simulink model "testrig_half_car_spla_s2laf_au"  (R2023a)
settings: Solver=ode23t  StartTime=0.0  StopTime=192  MaxStep=0.05  RelTol=1e-3  AbsTol=1e-3  EnableMultiTasking=on
PostLoadFcn:
  | sm_car_load_vehicle_data(bdroot,'220');
  | 
  | Vehicle.Chassis.SuspA1.Linkage.Upper_Arm_to_Subframe.class.Value  = 'Rigid_1Rev';
  | Vehicle.Chassis.SuspA1.Linkage.LowerArmF_to_Subframe.class.Value  = 'Rigid_UJ';
  | Vehicle.Chassis.SuspA1.Linkage.LowerArmR_to_Subframe.class.Value  = 'Rigid_UJ';
  | Vehicle.Chassis.SuspA1.AntiRollBar.SubframeConnection.class.Value = 'Rigid_1Rev';
  | 
  | Maneuver = sm_car_maneuverdata_knc(0.22,-0.15,0.01,1.0,0.10,500,1200,1200);
  | Vehicle = sm_car_vehcfg_checkConfig(Vehicle);
  | Visual = sm_car_param_visual('default');
undefined symbols (not defined in the file or in its folder): X, Y, Z
libraries: sm_lib x14, sm_car_testrig_utilities_lib x4, nesl_utility x4, fl_lib x4, Damper_Element x2, Linkage_SpLA_S2LAF_AU x2, Spring_Element x2, Suspension_Utilities x2, AntiRollBar_Droplink_Rod x1
CloseFcn:
  | clear simlog_sm_car_testrig_quarter_car
  | clear logsout_sm_car_testrig_quarter_car
Description:
  | Half Car Testrig, Pullrod
  | 
  | Copyright 2021-2024 The MathWorks, Inc.
settings Model: Creator=smiller  LastModifiedBy=smiller
settings SolverCC: AutoScaleAbsTol=off  AlgebraicLoopSolver=TrustRegion
settings DataIOCC: LimitDataPoints=on  MaxDataPoints=10000  ReturnWorkspaceOutputs=off  SignalLoggingName=logsout_sm_car_testrig_quarter_car
settings OptimizationCC: LifeSpan=inf
settings DebuggingCC: UnconnectedInputMsg=warning  UnconnectedOutputMsg=warning  UnconnectedLineMsg=warning  AllowSymbolicDim=off  SFUnexpectedBacktrackingDiag=warning  SFNoUnconditionalDefaultTransitionDiag=warning  SFExecutionAtInitializationDiag=none  ArithmeticOperatorsInVariantConditions=warning
settings ModelReferenceCC: EnableRefExpFcnMdlSchedulingChecks=on
settings SFSimCC: SimUseLocalCustomCode=off  CustomCodeUndefinedFunction=UseInterfaceOnly
settings RTWCC: RTWUseLocalCustomCode=off
settings CodeAppCC: StateflowObjectComments=on
settings GRTTargetCC: TargetLangStandard=C89/C90 (ANSI)
settings ConfigComp: CovMetricSettings=dw  CovSaveCumulativeToWorkspaceVar=on  CovSaveSingleToWorkspaceVar=on  CovExternalEMLEnable=off  CovSFcnEnable=off
settings SimscapeCC: SimscapeLogType=all  SimscapeLogSimulationStatistics=on  SimscapeLogName=simlog_sm_car_testrig_quarter_car  SimscapeLogLimitData=off  SimscapeLogDataHistory=10000  SimscapeOperatingPoint=op
settings DiagnosticsConfigSet: SimMechanicsUnconnectedFramePorts=none
settings ExplorerConfigSet: InternalSimMechanicsExplorerSettings="<ExplorerConfiguration><canonicalview>default</canonicalview><AnimationSetting><BasePlaybackSpeed>1.0</BasePlaybackSpeed><PlaybackSpeedFactor>16.0</PlaybackSpeedFactor></AnimationSetting><TilePanel><TileInfo><Tiles Columns=\"1\" Count=\"1\" Rows=\"1\"><Column Weight=\"1\"/><Row Weight=\"1\"/><Tile Height=\"1\" Width=\"1\" X=\"0\" Y=\"0\"/></Tiles></TileInfo><SceneInfo><SceneViewer><BGColor><R>1</R><G>1</G><B>1</B></BGColor><Camera><DoPerspective>off</DoPerspective><Position><X>0.571928528858414942</X><Y>-0.579111562749420217</Y><Z>0.83606068842340453</Z></Position><Center><X>-0.00542174033121090027</X><Y>-0.00176129355979437463</Y><Z>0.258710419233778688</Z></Center><Up><X>-0.408248290463863073</X><Y>0.408248290463863073</Y><Z>0.816496580927726145</Z></Up><ViewLimDist>1</ViewLimDist><YLim>0.718679582981457732</YLim><XLim>0.891323281686500546</XLim></Camera></SceneViewer></SceneInfo></TilePanel><MechEditorPanel><Cameras/><GfxPanelCameraMap/><VideoCreator><PlaybackSpeedRatio>1.0</PlaybackSpeedRatio><FrameRate>30</FrameRate><VideoFormat>Motion JPEG AVI</VideoFormat><FrameSize>auto</FrameSize></VideoCreator></MechEditorPanel></ExplorerConfiguration>"

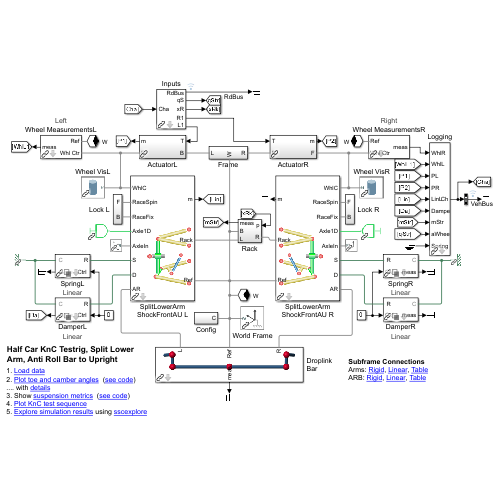
[thumbnail: Simulink's stored preview of the top-level diagram]
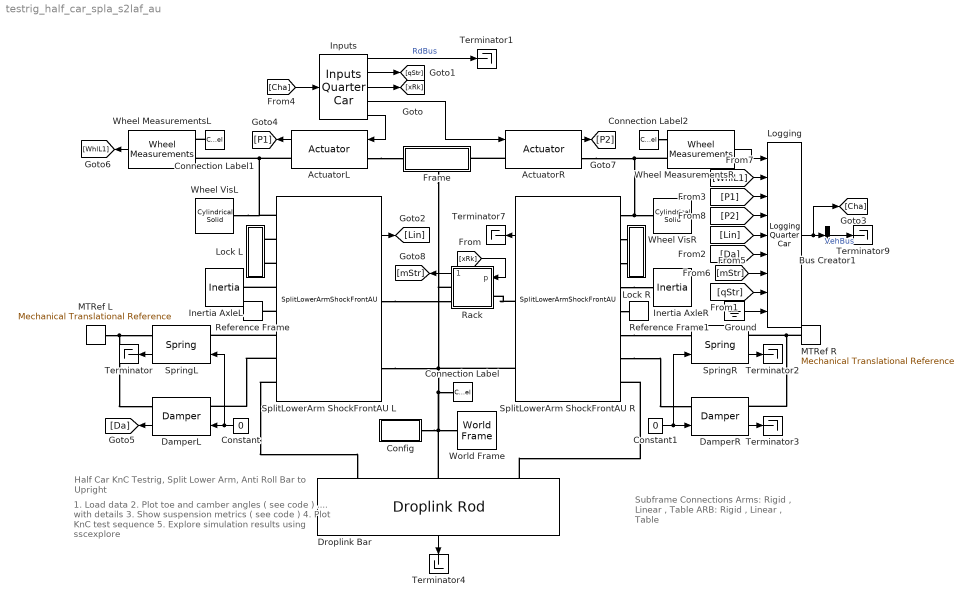
== system testrig_half_car_spla_s2laf_au ==
  note: Subframe Connections
      | Arms: Rigid , Linear , Table
      | ARB: Rigid , Linear , Table
  note: Half Car KnC Testrig, Split Lower
      | Arm, Anti Roll Bar to Upright
  note: 1. Load data
      | 2. Plot toe and camber angles ( see code )
      | .... with details
      | 3. Show suspension metrics ( see code )
      | 4. Plot KnC test sequence
      | 5. Explore simulation results using sscexplore
  ActuatorL : sm_car_testrig_utilities_lib/Actuator  SystemSampleTime=-1  VariantActivationTime=update diagram  Latency=0  AutoFrameSizeCalculation=off
  ActuatorR : sm_car_testrig_utilities_lib/Actuator  SystemSampleTime=-1  VariantActivationTime=update diagram  Latency=0  AutoFrameSizeCalculation=off
  Bus Creator1 : BusCreator  Inputs=1
  Config : Subsystem
  Connection Label : ConnectionLabel  Label=W
  Connection Label1 : ConnectionLabel  Label=W
  Connection Label2 : ConnectionLabel  Label=W
  Constant : Constant  Value=0
  Constant1 : Constant  Value=0
  DamperL : Damper_Element/Damper  VariantControl=Variant1  LabelModeActiveChoice=Linear  Damper=Vehicle.Chassis.Damper.Axle1  VariantLabel=Vehicle.Chassis.Damper.Axle1.class.Value
      settings: AttributesFormatString=%<ActiveVariant>
  DamperR : Damper_Element/Damper  VariantControl=Variant1  LabelModeActiveChoice=Linear  Damper=Vehicle.Chassis.Damper.Axle1  VariantLabel=Vehicle.Chassis.Damper.Axle1.class.Value
      settings: AttributesFormatString=%<ActiveVariant>
  Droplink Bar : AntiRollBar_Droplink_Rod/Droplink Rod  VariantControl=Variant1  hp_rod=Vehicle.Chassis.SuspA1.AntiRollBar.sSuspension.Value  hp_out=Vehicle.Chassis.SuspA1.AntiRollBar.sOutboard.Value  hp_in=Vehicle.Chassis.SuspA1.AntiRollBar.sInboard.Value  hp_mount_subframe=Vehicle.Chassis.SuspA1.AntiRollBar.sMount.Value  rotYAxis=Vehicle.Chassis.SuspA1.AntiRollBar.qUniversal.Value  SubframeConnection=Vehicle.Chassis.SuspA1.AntiRollBar.SubframeConnection  k=Vehicle.Chassis.SuspA1.AntiRollBar.k.Value  d=Vehicle.Chassis.SuspA1.AntiRollBar.d.Value  m=Vehicle.Chassis.SuspA1.AntiRollBar.m.Value  clr_solid=Visual.AntiRollBar.clr  opc_solid=Visual.part.opc  rad_solid=Visual.AntiRollBar.rad  clr_hp=Visual.hp.clr  opc_hp=Visual.hp.opc  rad_hp=Visual.hp.rad
  Frame : Subsystem
      settings: PortSchema="{\"entries\":[{\"content\":{\"sides\":[{\"content\":{\"connectorIds\":[\"LConn1\"]},\"type\":\"ConnectorPlacement.EquallySpacedRectSide\",\"uuid\":\"4d1860d1-8382-4b55-85c2-09349d56bb16\"},{\"content\":{\"connectorIds\":[\"RConn1\"],\"side\":\"RIGHT\"},\"type\":\"ConnectorPlacement.EquallySpacedRectSide\",\"uuid\":\"4e90683f-4b1a-48f4-aa4c-ab416257a32f\"},{\"content\":{\"connectorIds\":[],\"side\":\"TOP\"},\"type\":\"ConnectorPlacement.EquallySpacedRectSide\",\"uuid\":\"73ac831e-e43d-4cda-a295-19295eab84b4\"},{\"content\":{\"connectorIds\":[\"RConn2\"],\"side\":\"BOTTOM\"},\"type\":\"ConnectorPlacement.EquallySpacedRectSide\",\"uuid\":\"24788d71-0cf9-496d-9e47-2bd8b288be51\"}]},\"type\":\"ConnectorPlacement.EquallySpacedConnector\",\"uuid\":\"859ec081-8f6e-43e9-9a98-d438cbc0fcb8\"}],\"packageUris\":[\"http://schema.mathworks.com/mf0/Connector/R2020b\"],\"version\":\"1.0\"}"
  Ground : Ground
  Inertia AxleL : fl_lib/Mechanical/Rotational Elements/Inertia  inertia=0.01 kg*m^2  num_ports=foundation.enum.numPorts2.one  w_specify=on  w_priority=None  w=0 rad/s  w_nominal_specify=off  w_nominal_unit=rad/s  w_nominal_value=1  t_specify=off  t_priority=None  t=0 N*m  t_nominal_specify=off  t_nominal_unit=N*m  t_nominal_value=1
  Inertia AxleR : fl_lib/Mechanical/Rotational Elements/Inertia  inertia=0.01 kg*m^2  num_ports=foundation.enum.numPorts2.one  w_specify=on  w_priority=None  w=0 rad/s  w_nominal_specify=off  w_nominal_unit=rad/s  w_nominal_value=1  t_specify=off  t_priority=None  t=0 N*m  t_nominal_specify=off  t_nominal_unit=N*m  t_nominal_value=1
  Inputs : sm_car_testrig_utilities_lib/Inputs Quarter Car  popup_steering_input=On
  Lock L : Subsystem
  Lock R : Subsystem
  Logging : sm_car_testrig_utilities_lib/Logging Quarter Car
  MTRef L : fl_lib/Mechanical/Translational Elements/Mechanical Translational Reference
  MTRef R : fl_lib/Mechanical/Translational Elements/Mechanical Translational Reference
  Rack : Subsystem
  Reference Frame : sm_lib/Frames and Transforms/Reference Frame
  Reference Frame1 : sm_lib/Frames and Transforms/Reference Frame
  SplitLowerArm ShockFrontAU L : Linkage_SpLA_S2LAF_AU/SplitLowerArmShockFrontAU  VariantControl=SplitLowerArmShockFront  popup_leftRight=Left  hp_in_f_ua=Vehicle.Chassis.SuspA1.Linkage.UpperWishbone.sInboardF.Value  hp_in_r_ua=Vehicle.Chassis.SuspA1.Linkage.UpperWishbone.sInboardR.Value  hp_out_ua=Vehicle.Chassis.SuspA1.Linkage.UpperWishbone.sOutboard.Value  hp_in_f_la=Vehicle.Chassis.SuspA1.Linkage.LowerArmF.sInboard.Value  hp_in_r_la=Vehicle.Chassis.SuspA1.Linkage.LowerArmR.sInboard.Value  hp_out_f_la=Vehicle.Chassis.SuspA1.Linkage.LowerArmF.sOutboard.Value  hp_out_r_la=Vehicle.Chassis.SuspA1.Linkage.LowerArmR.sOutboard.Value  hp_upr_cg=Vehicle.Chassis.SuspA1.Linkage.Upright.sCG.Value  hp_upr_wc=Vehicle.Chassis.SuspA1.Linkage.Upright.sWheelCentre.Value  hp_upr_arb=Vehicle.Chassis.SuspA1.Linkage.Upright.sARB.Value  hp_in_rod=Vehicle.Chassis.SuspA1.Linkage.TrackRod.sInboard.Value  hp_upr_rod=Vehicle.Chassis.SuspA1.Linkage.TrackRod.sOutboard.Value  hp_spr_top=Vehicle.Chassis.SuspA1.Linkage.Shock.sTop.Value  hp_spr_bot=Vehicle.Chassis.SuspA1.Linkage.Shock.sBottom.Value  clr_hp=Visual.hp.clr  opc_hp=Visual.hp.opc  size_hp=Visual.hp.rad  Upper_Arm_to_Subframe=Vehicle.Chassis.SuspA1.Linkage.Upper_Arm_to_Subframe  ua_mass=Vehicle.Chassis.SuspA1.Linkage.UpperWishbone.m.Value  clr_ua=Visual.UpperArm.clr  opc_ua=Visual.part.opc  radius_ua=Visual.UpperArm.rad  LowerArmF_to_Subframe=Vehicle.Chassis.SuspA1.Linkage.LowerArmF_to_Subframe  LowerArmR_to_Subframe=Vehicle.Chassis.SuspA1.Linkage.LowerArmR_to_Subframe  laf_mass=Vehicle.Chassis.SuspA1.Linkage.LowerArmF.m.Value  lar_mass=Vehicle.Chassis.SuspA1.Linkage.LowerArmR.m.Value  clr_conn_la=Visual.hp.clr  opc_conn_la=Visual.hp.opc  size_conn_la=Visual.hp.rad  clr_laf=Visual.LowerArm.clr  opc_laf=Visual.part.opc  radius_laf=Visual.LowerArm.rad  clr_lar=Visual.LowerArm.clr  opc_lar=Visual.part.opc  radius_lar=Visual.LowerArm.rad  shock_pist_mass=Vehicle.Chassis.SuspA1.Linkage.Shock.mPiston.Value  shock_cyl_mass=Vehicle.Chassis.SuspA1.Linkage.Shock.mCylinder.Value  up_lim_bumpstop=Vehicle.Chassis.SuspA1.Linkage.Endstop.xMax.Value  low_lim_bumpstop=Vehicle.Chassis.SuspA1.Linkage.Endstop.xMin.Value  clr_conn_shock=Visual.hp.clr  opc_conn_shock=Visual.hp.opc  size_conn_shock=Visual.hp.rad  clr_shock_cyl=Visual.Shock.cyl.clr  opc_shock_cyl=Visual.part.opc  radius_shock_cyl=Visual.Shock.cyl.rad  clr_shock_piston=Visual.Shock.piston.clr  opc_shock_piston=Visual.part.opc  clr_shock_bumpstop=Visual.Shock.bumpstop.clr  opc_shock_bumpstop=Visual.part.opc  deadvol_len_shock_cyl=Visual.Shock.dead_length  piston_len_shock=Visual.Shock.piston.len  cyl_cap_len_shock=Visual.Shock.cap.len  bumpstop_len_shock=Visual.Shock.bumpstop.len  atoe=Vehicle.Chassis.SuspA1.Linkage.Upright.aToe.Value  acamber=Vehicle.Chassis.SuspA1.Linkage.Upright.aCamber.Value  upr_mass=Vehicle.Chassis.SuspA1.Linkage.Upright.m.Value  axle_len=Vehicle.Chassis.SuspA1.Linkage.Upright.xAxle.Value  axle_whlc_to_bearing=Vehicle.Chassis.SuspA1.Linkage.Upright.xWCtoBearing.Value  axle_mass=Vehicle.Chassis.SuspA1.Linkage.Upright.mAxle.Value  clr_conn_upr=Visual.hp.clr  opc_conn_upr=Visual.hp.opc  size_conn_upr=Visual.hp.rad  clr_upr=Visual.Upright.clr  opc_upr=Visual.part.opc  radius_upr=Visual.Upright.rad  clr_axle=Visual.Axle.clr  opc_axle=Visual.part.opc  radius_axle=Visual.Axle.rad  rod_mass=Vehicle.Chassis.SuspA1.Linkage.TrackRod.m.Value  clr_conn_rod=Visual.hp.clr  opc_conn_rod=Visual.hp.opc  size_conn_rod=Visual.hp.rad  clr_rod=Visual.TrackRod.clr  opc_rod=Visual.part.opc  radius_rod=Visual.TrackRod.rad  whl_init_spd_lr=Init.Axle1.nWheel.Value
  SplitLowerArm ShockFrontAU R : Linkage_SpLA_S2LAF_AU/SplitLowerArmShockFrontAU  VariantControl=SplitLowerArmShockFront  popup_leftRight=Right  hp_in_f_ua=Vehicle.Chassis.SuspA1.Linkage.UpperWishbone.sInboardF.Value  hp_in_r_ua=Vehicle.Chassis.SuspA1.Linkage.UpperWishbone.sInboardR.Value  hp_out_ua=Vehicle.Chassis.SuspA1.Linkage.UpperWishbone.sOutboard.Value  hp_in_f_la=Vehicle.Chassis.SuspA1.Linkage.LowerArmF.sInboard.Value  hp_in_r_la=Vehicle.Chassis.SuspA1.Linkage.LowerArmR.sInboard.Value  hp_out_f_la=Vehicle.Chassis.SuspA1.Linkage.LowerArmF.sOutboard.Value  hp_out_r_la=Vehicle.Chassis.SuspA1.Linkage.LowerArmR.sOutboard.Value  hp_upr_cg=Vehicle.Chassis.SuspA1.Linkage.Upright.sCG.Value  hp_upr_wc=Vehicle.Chassis.SuspA1.Linkage.Upright.sWheelCentre.Value  hp_upr_arb=Vehicle.Chassis.SuspA1.Linkage.Upright.sARB.Value  hp_in_rod=Vehicle.Chassis.SuspA1.Linkage.TrackRod.sInboard.Value  hp_upr_rod=Vehicle.Chassis.SuspA1.Linkage.TrackRod.sOutboard.Value  hp_spr_top=Vehicle.Chassis.SuspA1.Linkage.Shock.sTop.Value  hp_spr_bot=Vehicle.Chassis.SuspA1.Linkage.Shock.sBottom.Value  clr_hp=Visual.hp.clr  opc_hp=Visual.hp.opc  size_hp=Visual.hp.rad  Upper_Arm_to_Subframe=Vehicle.Chassis.SuspA1.Linkage.Upper_Arm_to_Subframe  ua_mass=Vehicle.Chassis.SuspA1.Linkage.UpperWishbone.m.Value  clr_ua=Visual.UpperArm.clr  opc_ua=Visual.part.opc  radius_ua=Visual.UpperArm.rad  LowerArmF_to_Subframe=Vehicle.Chassis.SuspA1.Linkage.LowerArmF_to_Subframe  LowerArmR_to_Subframe=Vehicle.Chassis.SuspA1.Linkage.LowerArmR_to_Subframe  laf_mass=Vehicle.Chassis.SuspA1.Linkage.LowerArmF.m.Value  lar_mass=Vehicle.Chassis.SuspA1.Linkage.LowerArmR.m.Value  clr_conn_la=Visual.hp.clr  opc_conn_la=Visual.hp.opc  size_conn_la=Visual.hp.rad  clr_laf=Visual.LowerArm.clr  opc_laf=Visual.part.opc  radius_laf=Visual.LowerArm.rad  clr_lar=Visual.LowerArm.clr  opc_lar=Visual.part.opc  radius_lar=Visual.LowerArm.rad  shock_pist_mass=Vehicle.Chassis.SuspA1.Linkage.Shock.mPiston.Value  shock_cyl_mass=Vehicle.Chassis.SuspA1.Linkage.Shock.mCylinder.Value  up_lim_bumpstop=Vehicle.Chassis.SuspA1.Linkage.Endstop.xMax.Value  low_lim_bumpstop=Vehicle.Chassis.SuspA1.Linkage.Endstop.xMin.Value  clr_conn_shock=Visual.hp.clr  opc_conn_shock=Visual.hp.opc  size_conn_shock=Visual.hp.rad  clr_shock_cyl=Visual.Shock.cyl.clr  opc_shock_cyl=Visual.part.opc  radius_shock_cyl=Visual.Shock.cyl.rad  clr_shock_piston=Visual.Shock.piston.clr  opc_shock_piston=Visual.part.opc  clr_shock_bumpstop=Visual.Shock.bumpstop.clr  opc_shock_bumpstop=Visual.part.opc  deadvol_len_shock_cyl=Visual.Shock.dead_length  piston_len_shock=Visual.Shock.piston.len  cyl_cap_len_shock=Visual.Shock.cap.len  bumpstop_len_shock=Visual.Shock.bumpstop.len  atoe=Vehicle.Chassis.SuspA1.Linkage.Upright.aToe.Value  acamber=Vehicle.Chassis.SuspA1.Linkage.Upright.aCamber.Value  upr_mass=Vehicle.Chassis.SuspA1.Linkage.Upright.m.Value  axle_len=Vehicle.Chassis.SuspA1.Linkage.Upright.xAxle.Value  axle_whlc_to_bearing=Vehicle.Chassis.SuspA1.Linkage.Upright.xWCtoBearing.Value  axle_mass=Vehicle.Chassis.SuspA1.Linkage.Upright.mAxle.Value  clr_conn_upr=Visual.hp.clr  opc_conn_upr=Visual.hp.opc  size_conn_upr=Visual.hp.rad  clr_upr=Visual.Upright.clr  opc_upr=Visual.part.opc  radius_upr=Visual.Upright.rad  clr_axle=Visual.Axle.clr  opc_axle=Visual.part.opc  radius_axle=Visual.Axle.rad  rod_mass=Vehicle.Chassis.SuspA1.Linkage.TrackRod.m.Value  clr_conn_rod=Visual.hp.clr  opc_conn_rod=Visual.hp.opc  size_conn_rod=Visual.hp.rad  clr_rod=Visual.TrackRod.clr  opc_rod=Visual.part.opc  radius_rod=Visual.TrackRod.rad  whl_init_spd_lr=Init.Axle1.nWheel.Value
  SpringL : Spring_Element/Spring  VariantControl=Variant1  LabelModeActiveChoice=Linear  Spring=Vehicle.Chassis.Spring.Axle1  VariantLabel=Vehicle.Chassis.Spring.Axle1.class.Value
      settings: AttributesFormatString=%<ActiveVariant>
  SpringR : Spring_Element/Spring  VariantControl=Variant1  LabelModeActiveChoice=Linear  Spring=Vehicle.Chassis.Spring.Axle1  VariantLabel=Vehicle.Chassis.Spring.Axle1.class.Value
      settings: AttributesFormatString=%<ActiveVariant>
  Terminator{,1..4,7,9} (7 alike) : Terminator
  Wheel MeasurementsL : Suspension_Utilities/Wheel Measurements  popup_leftRight=Left
      settings: AttributesFormatString=%<popup_leftRight>
  Wheel MeasurementsR : Suspension_Utilities/Wheel Measurements  popup_leftRight=Right
      settings: AttributesFormatString=%<popup_leftRight>
  Wheel VisL : sm_lib/Body Elements/Cylindrical Solid  GraphicAmbientColor=[0.15 0.15 0.15 1.0]  BasedOnType=Mass  CenterOfMass=[0 0 0]  CenterOfMassUnits=m  GraphicDiffuseColor=[0.5 0.5 0.5]  CylinderLength=Vehicle.Chassis.TireA1.tire_radius.Value*0.6  CylinderLengthUnits=m  CylinderRadius=Vehicle.Chassis.TireA1.tire_radius.Value  CylinderRadiusUnits=m  Density=1000  DensityUnits=kg/m^3  DoExposeReferenceFrame=on  GraphicEmissiveColor=[0.0 0.0 0.0 1.0]  ExportEntireGeometry=off  SerializedFrames=<Frames/>  MarkerShape=Sphere  MarkerSize=10  GraphicType=FromGeometry  InertiaType=CalculateFromGeometry  Mass=Vehicle.Chassis.TireA1.Mass.Value  MassUnits=kg  MomentsOfInertia=[1 1 1]  MomentsOfInertiaUnits=kg*m^2  GraphicOpacity=0.3  ProductsOfInertia=[0 0 0]  ProductsOfInertiaUnits=kg*m^2  GraphicShininess=75  GraphicSpecularColor=[0.5 0.5 0.5 1.0]  GraphicVisPropType=SimpleVisualProperties
  Wheel VisR : sm_lib/Body Elements/Cylindrical Solid  GraphicAmbientColor=[0.15 0.15 0.15 1.0]  BasedOnType=Mass  CenterOfMass=[0 0 0]  CenterOfMassUnits=m  GraphicDiffuseColor=[0.5 0.5 0.5]  CylinderLength=Vehicle.Chassis.TireA1.tire_radius.Value*0.6  CylinderLengthUnits=m  CylinderRadius=Vehicle.Chassis.TireA1.tire_radius.Value  CylinderRadiusUnits=m  Density=1000  DensityUnits=kg/m^3  DoExposeReferenceFrame=on  GraphicEmissiveColor=[0.0 0.0 0.0 1.0]  ExportEntireGeometry=off  SerializedFrames=<Frames/>  MarkerShape=Sphere  MarkerSize=10  GraphicType=FromGeometry  InertiaType=CalculateFromGeometry  Mass=Vehicle.Chassis.TireA1.Mass.Value  MassUnits=kg  MomentsOfInertia=[1 1 1]  MomentsOfInertiaUnits=kg*m^2  GraphicOpacity=0.3  ProductsOfInertia=[0 0 0]  ProductsOfInertiaUnits=kg*m^2  GraphicShininess=75  GraphicSpecularColor=[0.5 0.5 0.5 1.0]  GraphicVisPropType=SimpleVisualProperties
  World Frame : sm_lib/Frames and Transforms/World Frame
  wires:
  DamperL/1 -> [Da]
  Constant/1 -> SpringL/1, DamperL/1
  SpringL/1 -> Terminator/1
  [xRk] -> Rack/1(p)
  SpringR/1 -> Terminator2/1
  Constant1/1 -> SpringR/1, DamperR/1
  DamperR/1 -> Terminator3/1
  Droplink Bar/1 -> Terminator4/1
  ActuatorR/1 -> [P2]
  SplitLowerArm ShockFrontAU L/1 -> [Lin]
  SplitLowerArm ShockFrontAU R/1 -> Terminator7/1
  Wheel MeasurementsL/1 -> [WhlL1]
  [P1] -> Logging/3
  [Lin] -> Logging/5
  [WhlL1] -> Logging/2
  Bus Creator1/1 -> Terminator9/1  "VehBus"
  ActuatorL/1 -> [P1]
  [Cha] -> Inputs/1
  Inputs/5 -> ActuatorL/1
  Inputs/4 -> ActuatorR/1
  Inputs/2 -> [qStr]
  Inputs/3 -> [xRk]
  Inputs/1 -> Terminator1/1  "RdBus"
  Wheel MeasurementsR/1 -> Logging/1
  Logging/1 -> [Cha], Bus Creator1/1
  [Da] -> Logging/6
  [mStr] -> Logging/7
  [qStr] -> Logging/8
  Ground/1 -> Logging/9
  [P2] -> Logging/4
  Rack/1(meas) -> [mStr]
  connections:
  Wheel VisL/RConn1 -- SplitLowerArm ShockFrontAU L/LConn1 -- ActuatorL/RConn1 -- Wheel MeasurementsL/LConn2
  MTRef L/LConn1 -- SpringL/RConn1 -- DamperL/RConn1
  Config/RConn1 -- Droplink Bar/LConn2 -- World Frame/RConn1 -- Frame/RConn2 -- Rack/RConn1 -- SplitLowerArm ShockFrontAU R/RConn2 -- SplitLowerArm ShockFrontAU L/RConn2 -- Connection Label/LConn1
  SplitLowerArm ShockFrontAU L/LConn6 -- SpringL/LConn1
  SplitLowerArm ShockFrontAU L/LConn4 -- Inertia AxleL/LConn1
  SplitLowerArm ShockFrontAU L/LConn5 -- Reference Frame/RConn1
  SplitLowerArm ShockFrontAU L/LConn7 -- DamperL/LConn1
  SplitLowerArm ShockFrontAU L/RConn1 -- Rack/RConn2
  ActuatorR/RConn1 -- SplitLowerArm ShockFrontAU R/LConn1 -- Wheel VisR/RConn1 -- Wheel MeasurementsR/LConn2
  MTRef R/LConn1 -- DamperR/RConn1 -- SpringR/RConn1
  SplitLowerArm ShockFrontAU R/LConn4 -- Inertia AxleR/LConn1
  SplitLowerArm ShockFrontAU R/LConn6 -- SpringR/LConn1
  SplitLowerArm ShockFrontAU R/LConn5 -- Reference Frame1/RConn1
  SplitLowerArm ShockFrontAU R/LConn7 -- DamperR/LConn1
  SplitLowerArm ShockFrontAU L/LConn8 -- Droplink Bar/LConn1
  SplitLowerArm ShockFrontAU R/RConn1 -- Rack/LConn1
  SplitLowerArm ShockFrontAU R/LConn2 -- Lock R/LConn1
  SplitLowerArm ShockFrontAU R/LConn3 -- Lock R/LConn2
  SplitLowerArm ShockFrontAU L/LConn2 -- Lock L/LConn1
  SplitLowerArm ShockFrontAU L/LConn3 -- Lock L/LConn2
  ActuatorL/LConn1 -- Frame/LConn1
  ActuatorR/LConn1 -- Frame/RConn1
  Connection Label1/LConn1 -- Wheel MeasurementsL/LConn1
  Droplink Bar/LConn3 -- SplitLowerArm ShockFrontAU R/LConn8
  Connection Label2/LConn1 -- Wheel MeasurementsR/LConn1

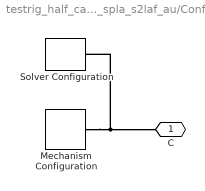
== system testrig_half_car_spla_s2laf_au/Config ==
  Mechanism Configuration : sm_lib/Utilities/Mechanism Configuration  UniformGravity=Constant  GravityVector=[0 0 -9.80665]  GravityVectorUnits=m/s^2  LinearizationDelta=0.001  JointModeTransitionNonlinearIterations=2
  Solver Configuration : nesl_utility/Solver Configuration  PhysicalDomain=network_engine_domain  SubClassName=solver  LeftPortType=input  RightPortType=generic  Tones=[]  Harmonics=[]  SimulateNoise=off  Profile=off  UseLocalSampling=off  EnableSwitchedLinearOptims=on  FrequencyDomain=off  UseCCode=off  RelTol=0.001  AbsTol=1e-06  MinStep=1e-09  ToWorkspace=off  RevertToSquareIcSolve=off  NumHomotopyIterations=100  PhasorMode=off  PhasorModeNumHarmonics=1  ConsistencySolver=NEWTON_FTOL  IndexReductionMethod=DerivativeReplacement  DoDC=off  ResidualTolerance=1e-09  ConsistencyTolSource=GLOBAL  ConsistencyAbsTol=0.001  ConsistencyRelTol=0.001  ConsistencyTolFactor=0.001  UseLocalSolver=off  LocalSolverChoice=NE_BACKWARD_EULER_ADVANCER  ResolveIndetEquations=on  FunctionEvalNumThread=1  LocalSolverSampleTime=0.001  DoFixedCost=off  MaxNonlinIter=3  MaxModeIter=2  ComputeImpulses=off  ImpulseIterations=2  LinearAlgebra=Sparse  LinearAlgebraNumThread=0  EquationFormulation=NE_TIME_EF  DelaysMemoryBudget=1024  AutomaticFiltering=on  FilteringTimeConstant=0.001  PartitionStorageMethod=AS_NEEDED  PartitionMemoryBudget=1024  PartitionMethod=FAST
  C : PMIOPort  Side=Right
  connections:
  Mechanism Configuration/RConn1 -- Solver Configuration/RConn1 -- C/RConn1

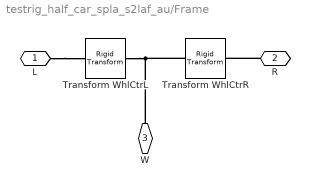
== system testrig_half_car_spla_s2laf_au/Frame ==
  Transform WhlCtrL : sm_lib/Frames and Transforms/Rigid Transform  TranslationMethod=Cartesian  TranslationStandardOffset=0  TranslationStandardOffsetUnits=m  TranslationStandardAxis=+Z  TranslationCartesianOffset=Vehicle.Chassis.SuspA1.Linkage.Upright.sWheelCentre.Value  TranslationCartesianOffsetUnits=m  TranslationROffset=0  TranslationROffsetUnits=m  TranslationZOffset=0  TranslationZOffsetUnits=m  TranslationThetaOffset=0  TranslationThetaOffsetUnits=deg  RotationMethod=None  RotationAngleUnits=deg  RotationStandardAxis=+Z  RotationAngle=0.0  RotationArbitraryAxis=[0 0 1]  FollAlignAxisA=+X  BaseAlignAxisA=+Y  FollAlignAxisB=+Y  BaseAlignAxisB=+Z  RotationSequenceAxes=FollowerAxes  RotationSequence=XYX  RotationSequenceAngles=[0 0 0]  RotationSequenceAnglesUnits=deg  RotationMatrix=[1 0 0; 0 1 0; 0 0 1]  Quaternion=[1 0 0 0]
  Transform WhlCtrR : sm_lib/Frames and Transforms/Rigid Transform  TranslationMethod=Cartesian  TranslationStandardOffset=0  TranslationStandardOffsetUnits=m  TranslationStandardAxis=+Z  TranslationCartesianOffset=Vehicle.Chassis.SuspA1.Linkage.Upright.sWheelCentre.Value.*[1 -1 1]  TranslationCartesianOffsetUnits=m  TranslationROffset=0  TranslationROffsetUnits=m  TranslationZOffset=0  TranslationZOffsetUnits=m  TranslationThetaOffset=0  TranslationThetaOffsetUnits=deg  RotationMethod=None  RotationAngleUnits=deg  RotationStandardAxis=+Z  RotationAngle=0.0  RotationArbitraryAxis=[0 0 1]  FollAlignAxisA=+X  BaseAlignAxisA=+Y  FollAlignAxisB=+Y  BaseAlignAxisB=+Z  RotationSequenceAxes=FollowerAxes  RotationSequence=XYX  RotationSequenceAngles=[0 0 0]  RotationSequenceAnglesUnits=deg  RotationMatrix=[1 0 0; 0 1 0; 0 0 1]  Quaternion=[1 0 0 0]
  L : PMIOPort  Side=Left
  R : PMIOPort  Port=2  Side=Right
  W : PMIOPort  Port=3  Side=Right
  connections:
  R/RConn1 -- Transform WhlCtrR/RConn1
  L/RConn1 -- Transform WhlCtrL/RConn1
  W/RConn1 -- Transform WhlCtrL/LConn1 -- Transform WhlCtrR/LConn1

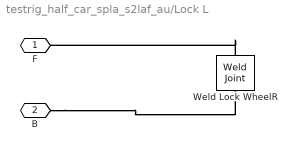
== system testrig_half_car_spla_s2laf_au/Lock L ==
  Weld Lock WheelR : sm_lib/Joints/Weld Joint  JointMode=Normal  SenseConstraintForce=off  SenseConstraintForceX=off  SenseConstraintForceY=off  SenseConstraintForceZ=off  SenseConstraintTorque=off  SenseConstraintTorqueX=off  SenseConstraintTorqueY=off  SenseConstraintTorqueZ=off  SenseTotalForce=off  SenseTotalForceX=off  SenseTotalForceY=off  SenseTotalForceZ=off  SenseTotalTorque=off  SenseTotalTorqueX=off  SenseTotalTorqueY=off  SenseTotalTorqueZ=off  CompositeWrenchDir=FollowerOnBase  CompositeWrenchFrame=BaseFrame
  F : PMIOPort  Side=Left
  B : PMIOPort  Port=2  Side=Left
  connections:
  B/RConn1 -- Weld Lock WheelR/LConn1
  Weld Lock WheelR/RConn1 -- F/RConn1

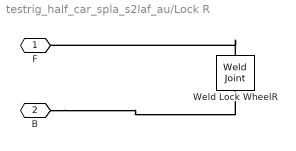
== system testrig_half_car_spla_s2laf_au/Lock R ==
  Weld Lock WheelR : sm_lib/Joints/Weld Joint  JointMode=Normal  SenseConstraintForce=off  SenseConstraintForceX=off  SenseConstraintForceY=off  SenseConstraintForceZ=off  SenseConstraintTorque=off  SenseConstraintTorqueX=off  SenseConstraintTorqueY=off  SenseConstraintTorqueZ=off  SenseTotalForce=off  SenseTotalForceX=off  SenseTotalForceY=off  SenseTotalForceZ=off  SenseTotalTorque=off  SenseTotalTorqueX=off  SenseTotalTorqueY=off  SenseTotalTorqueZ=off  CompositeWrenchDir=FollowerOnBase  CompositeWrenchFrame=BaseFrame
  F : PMIOPort  Side=Left
  B : PMIOPort  Port=2  Side=Left
  connections:
  Weld Lock WheelR/RConn1 -- F/RConn1
  B/RConn1 -- Weld Lock WheelR/LConn1

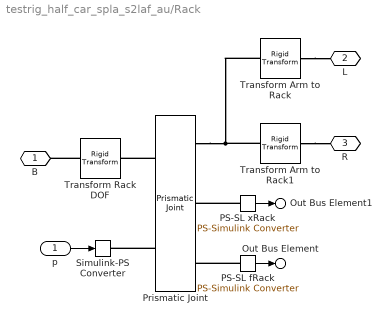
== system testrig_half_car_spla_s2laf_au/Rack ==
  p : Inport
  PS-SL fRack : nesl_utility/PS-Simulink Converter  PhysicalDomain=network_engine_domain  SubClassName=ps_output  LeftPortType=input  RightPortType=output  PseudoPeriodic=off  Frequencies=[]  VectorFormat=1-D array  Unit=1  AffineConversion=off
  PS-SL xRack : nesl_utility/PS-Simulink Converter  PhysicalDomain=network_engine_domain  SubClassName=ps_output  LeftPortType=input  RightPortType=output  PseudoPeriodic=off  Frequencies=[]  VectorFormat=1-D array  Unit=1  AffineConversion=off
  Prismatic Joint : sm_lib/Joints/Prismatic Joint  JointMode=Normal  SenseConstraintForce=off  SenseConstraintForceX=off  SenseConstraintForceY=off  SenseConstraintForceZ=off  SenseConstraintTorque=off  SenseConstraintTorqueX=off  SenseConstraintTorqueY=off  SenseConstraintTorqueZ=off  SenseTotalForce=off  SenseTotalForceX=off  SenseTotalForceY=off  SenseTotalForceZ=off  SenseTotalTorque=off  SenseTotalTorqueX=off  SenseTotalTorqueY=off  SenseTotalTorqueZ=off  CompositeWrenchDir=FollowerOnBase  CompositeWrenchFrame=BaseFrame  EquilibriumPosition=0  EquilibriumPositionUnits=m  SpringStiffness=0  SpringStiffnessUnits=N/m  DampingCoefficient=0  DampingCoefficientUnits=N/(m/s)  TorqueActuationMode=ComputedTorque  MotionActuationMode=InputMotion  SensePosition=on  SenseVelocity=off  SenseAcceleration=off  SenseTorqueForce=on  SenseLowerLimitTorqueForce=off  SenseUpperLimitTorqueForce=off  LowerLimitSpecify=off  LowerLimitBound=-1  LowerLimitBoundUnits=m  LowerLimitStiffness=1e6  LowerLimitStiffnessUnits=N/m  LowerLimitDamping=1e3  LowerLimitDampingUnits=N/(m/s)  LowerLimitTransitionRegionWidth=1e-4  LowerLimitTransitionRegionWidthUnits=m  UpperLimitSpecify=off  UpperLimitBound=1  UpperLimitBoundUnits=m  UpperLimitStiffness=1e6  UpperLimitStiffnessUnits=N/m  UpperLimitDamping=1e3  UpperLimitDampingUnits=N/(m/s)  UpperLimitTransitionRegionWidth=1e-4  UpperLimitTransitionRegionWidthUnits=m  PositionTargetSpecify=on  PositionTargetPriority=High  PositionTargetValue=0  PositionTargetValueUnits=m  VelocityTargetSpecify=off  VelocityTargetPriority=High  VelocityTargetValue=0  VelocityTargetValueUnits=m/s
  Simulink-PS Converter : nesl_utility/Simulink-PS Converter  PhysicalDomain=network_engine_domain  SubClassName=ps_input  LeftPortType=input  RightPortType=output  PseudoPeriodic=off  Frequencies=[]  NoiseDistribution=none  NoiseParameters=[]  Unit=m  AffineConversion=off  FilteringAndDerivatives=filter  SimscapeFilterOrder=2  InputFilterTimeConstant=0.1  UdotUserProvided=0
  Transform Arm to Rack : sm_lib/Frames and Transforms/Rigid Transform  TranslationMethod=Cartesian  TranslationStandardOffset=0  TranslationStandardOffsetUnits=m  TranslationStandardAxis=+Z  TranslationCartesianOffset=Vehicle.Chassis.SuspA1.Linkage.TrackRod.sInboard.Value.*[1 0 1]  TranslationCartesianOffsetUnits=m  TranslationROffset=0  TranslationROffsetUnits=m  TranslationZOffset=0  TranslationZOffsetUnits=m  TranslationThetaOffset=0  TranslationThetaOffsetUnits=deg  RotationMethod=StandardAxis  RotationAngleUnits=deg  RotationStandardAxis=+X  RotationAngle=90  RotationArbitraryAxis=[0 0 1]  FollAlignAxisA=+X  BaseAlignAxisA=+Y  FollAlignAxisB=+Y  BaseAlignAxisB=+Z  RotationSequenceAxes=FollowerAxes  RotationSequence=XYX  RotationSequenceAngles=[0 0 0]  RotationSequenceAnglesUnits=deg  RotationMatrix=[1 0 0; 0 1 0; 0 0 1]  Quaternion=[1 0 0 0]
  Transform Arm to Rack1 : sm_lib/Frames and Transforms/Rigid Transform  TranslationMethod=Cartesian  TranslationStandardOffset=0  TranslationStandardOffsetUnits=m  TranslationStandardAxis=+Z  TranslationCartesianOffset=Vehicle.Chassis.SuspA1.Linkage.TrackRod.sInboard.Value.*[1 0 1]  TranslationCartesianOffsetUnits=m  TranslationROffset=0  TranslationROffsetUnits=m  TranslationZOffset=0  TranslationZOffsetUnits=m  TranslationThetaOffset=0  TranslationThetaOffsetUnits=deg  RotationMethod=StandardAxis  RotationAngleUnits=deg  RotationStandardAxis=+X  RotationAngle=90  RotationArbitraryAxis=[0 0 1]  FollAlignAxisA=+X  BaseAlignAxisA=+Y  FollAlignAxisB=+Y  BaseAlignAxisB=+Z  RotationSequenceAxes=FollowerAxes  RotationSequence=XYX  RotationSequenceAngles=[0 0 0]  RotationSequenceAnglesUnits=deg  RotationMatrix=[1 0 0; 0 1 0; 0 0 1]  Quaternion=[1 0 0 0]
  Transform Rack DOF : sm_lib/Frames and Transforms/Rigid Transform  TranslationMethod=Cartesian  TranslationStandardOffset=0  TranslationStandardOffsetUnits=m  TranslationStandardAxis=+Z  TranslationCartesianOffset=Vehicle.Chassis.SuspA1.Linkage.TrackRod.sInboard.Value.*[1 0 1]  TranslationCartesianOffsetUnits=m  TranslationROffset=0  TranslationROffsetUnits=m  TranslationZOffset=0  TranslationZOffsetUnits=m  TranslationThetaOffset=0  TranslationThetaOffsetUnits=deg  RotationMethod=StandardAxis  RotationAngleUnits=deg  RotationStandardAxis=+X  RotationAngle=90  RotationArbitraryAxis=[0 0 1]  FollAlignAxisA=+X  BaseAlignAxisA=+Y  FollAlignAxisB=+Y  BaseAlignAxisB=+Z  RotationSequenceAxes=FollowerAxes  RotationSequence=XYX  RotationSequenceAngles=[0 0 0]  RotationSequenceAnglesUnits=deg  RotationMatrix=[1 0 0; 0 1 0; 0 0 1]  Quaternion=[1 0 0 0]
  B : PMIOPort  Side=Right
  L : PMIOPort  Port=2  Side=Right
  R : PMIOPort  Port=3  Side=Left
  Out Bus Element : Outport  VectorParamsAs1DForOutWhenUnconnected=off  PortName=meas  Element=FRack
  Out Bus Element1 : Outport  VectorParamsAs1DForOutWhenUnconnected=off  PortName=meas  Element=xRack
  wires:
  p/1 -> Simulink-PS Converter/1
  PS-SL xRack/1 -> Out Bus Element1/1
  PS-SL fRack/1 -> Out Bus Element/1
  connections:
  Prismatic Joint/LConn1 -- Transform Rack DOF/RConn1
  Prismatic Joint/LConn2 -- Simulink-PS Converter/RConn1
  Transform Arm to Rack/LConn1 -- L/RConn1
  Transform Arm to Rack/RConn1 -- Prismatic Joint/RConn1 -- Transform Arm to Rack1/RConn1
  Transform Rack DOF/LConn1 -- B/RConn1
  Transform Arm to Rack1/LConn1 -- R/RConn1
  PS-SL fRack/LConn1 -- Prismatic Joint/RConn3
  PS-SL xRack/LConn1 -- Prismatic Joint/RConn2
